simulink model "STC_Cepstral_Distance"  (Simulink 6.0)
settings: Solver=FixedStepDiscrete  SolverMode=SingleTasking  StartTime=0.0  StopTime=1  FixedStep=1/8000  RelTol=1e-3
libraries: dsplp x24, dspindex x16, dspbuff3 x8, dspsolvers x8, dspsrcs4 x6, dspsnks4 x4
settings Model: LastModifiedBy=Paulo

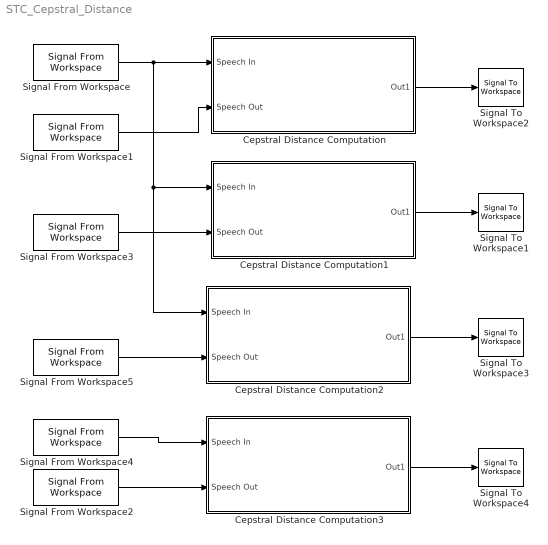
== system STC_Cepstral_Distance ==
  Cepstral Distance Computation : Subsystem
  Cepstral Distance Computation1 : Subsystem
  Cepstral Distance Computation2 : Subsystem
  Cepstral Distance Computation3 : Subsystem
  Signal From Workspace : dspsrcs4/Signal From Workspace  X=speech  Ts=1/8000  nsamps=160  OutputAfterFinalValue=Setting to zero
  Signal From Workspace1 : dspsrcs4/Signal From Workspace  X=speech1  Ts=1/8000  nsamps=160  OutputAfterFinalValue=Setting to zero
  Signal From Workspace2 : dspsrcs4/Signal From Workspace  X=speech3  Ts=1/8000  nsamps=160  OutputAfterFinalValue=Setting to zero
  Signal From Workspace3 : dspsrcs4/Signal From Workspace  X=speech2  Ts=1/8000  nsamps=160  OutputAfterFinalValue=Setting to zero
  Signal From Workspace4 : dspsrcs4/Signal From Workspace  X=residual  Ts=1/8000  nsamps=160  OutputAfterFinalValue=Setting to zero
  Signal From Workspace5 : dspsrcs4/Signal From Workspace  X=speech3  Ts=1/8000  nsamps=160  OutputAfterFinalValue=Setting to zero
  Signal To Workspace1 : dspsnks4/Signal To Workspace  VariableName=CD2  FrameMode=Concatenate frames (2-D array)
      settings: FixptAsFi=off
  Signal To Workspace2 : dspsnks4/Signal To Workspace  VariableName=CD1  FrameMode=Concatenate frames (2-D array)
      settings: FixptAsFi=off
  Signal To Workspace3 : dspsnks4/Signal To Workspace  VariableName=CD3  FrameMode=Concatenate frames (2-D array)
      settings: FixptAsFi=off
  Signal To Workspace4 : dspsnks4/Signal To Workspace  VariableName=CD4  FrameMode=Concatenate frames (2-D array)
      settings: FixptAsFi=off
  wires:
  Signal From Workspace/1 -> Cepstral Distance Computation/1(Speech In), Cepstral Distance Computation1/1(Speech In), Cepstral Distance Computation2/1(Speech In)
  Signal From Workspace1/1 -> Cepstral Distance Computation/2(Speech Out)
  Cepstral Distance Computation/1(Out1) -> Signal To Workspace2/1
  Signal From Workspace3/1 -> Cepstral Distance Computation1/2(Speech Out)
  Cepstral Distance Computation1/1(Out1) -> Signal To Workspace1/1
  Signal From Workspace5/1 -> Cepstral Distance Computation2/2(Speech Out)
  Cepstral Distance Computation2/1(Out1) -> Signal To Workspace3/1
  Signal From Workspace2/1 -> Cepstral Distance Computation3/2(Speech Out)
  Cepstral Distance Computation3/1(Out1) -> Signal To Workspace4/1
  Signal From Workspace4/1 -> Cepstral Distance Computation3/1(Speech In)

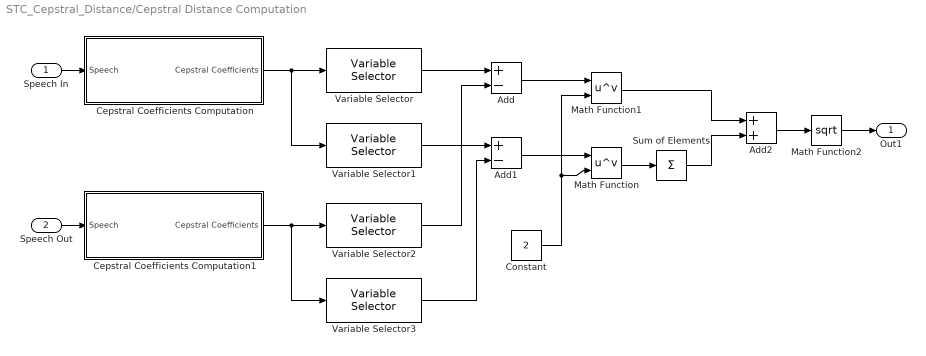
== system STC_Cepstral_Distance/Cepstral Distance Computation ==
  Speech In : Inport  Port=1  LatchInput=off
  Speech Out : Inport  Port=2  LatchInput=off
  Add : Sum  Inputs=+-  OutScaling=2^-10
  Add1 : Sum  Inputs=+-  OutScaling=2^-10
  Add2 : Sum  OutScaling=2^-10
  Cepstral Coefficients Computation : Subsystem
  Cepstral Coefficients Computation1 : Subsystem
  Constant : Constant  Value=2
  Math Function : Math  Operator=pow  SaturateOnIntegerOverflow=on
  Math Function1 : Math  Operator=pow  SaturateOnIntegerOverflow=on
  Math Function2 : Math  Operator=sqrt  SaturateOnIntegerOverflow=on
  Sum of Elements : Sum  Inputs=+  OutScaling=2^-10
  Variable Selector : dspindex/Variable Selector  rowsOrCols=Rows  IdxMode=Fixed  Elements=[1]  ZerOneIdxMode=One-based  errmode=Clip Index
  Variable Selector1 : dspindex/Variable Selector  rowsOrCols=Rows  IdxMode=Fixed  Elements=[2:21]  ZerOneIdxMode=One-based  errmode=Clip Index
  Variable Selector2 : dspindex/Variable Selector  rowsOrCols=Rows  IdxMode=Fixed  Elements=[1]  ZerOneIdxMode=One-based  errmode=Clip Index
  Variable Selector3 : dspindex/Variable Selector  rowsOrCols=Rows  IdxMode=Fixed  Elements=[2:21]  ZerOneIdxMode=One-based  errmode=Clip Index
  Out1 : Outport
  wires:
  Cepstral Coefficients Computation/1(Cepstral Coefficients) -> Variable Selector/1, Variable Selector1/1
  Cepstral Coefficients Computation1/1(Cepstral Coefficients) -> Variable Selector2/1, Variable Selector3/1
  Variable Selector/1 -> Add/1
  Variable Selector2/1 -> Add/2
  Variable Selector3/1 -> Add1/2
  Variable Selector1/1 -> Add1/1
  Add1/1 -> Math Function/1
  Constant/1 -> Math Function/2, Math Function1/2
  Math Function/1 -> Sum of Elements/1
  Add/1 -> Math Function1/1
  Sum of Elements/1 -> Add2/2
  Math Function1/1 -> Add2/1
  Add2/1 -> Math Function2/1
  Speech In/1 -> Cepstral Coefficients Computation/1(Speech)
  Math Function2/1 -> Out1/1
  Speech Out/1 -> Cepstral Coefficients Computation1/1(Speech)

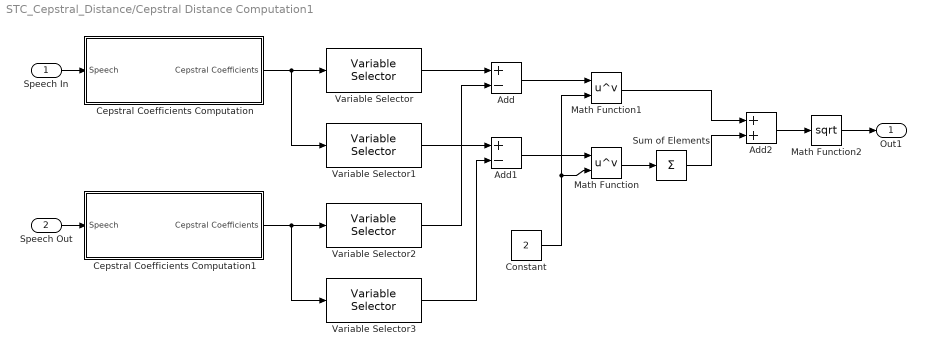
== system STC_Cepstral_Distance/Cepstral Distance Computation1 ==
  Speech In : Inport  Port=1  LatchInput=off
  Speech Out : Inport  Port=2  LatchInput=off
  Add : Sum  Inputs=+-  OutScaling=2^-10
  Add1 : Sum  Inputs=+-  OutScaling=2^-10
  Add2 : Sum  OutScaling=2^-10
  Cepstral Coefficients Computation : Subsystem
  Cepstral Coefficients Computation1 : Subsystem
  Constant : Constant  Value=2
  Math Function : Math  Operator=pow  SaturateOnIntegerOverflow=on
  Math Function1 : Math  Operator=pow  SaturateOnIntegerOverflow=on
  Math Function2 : Math  Operator=sqrt  SaturateOnIntegerOverflow=on
  Sum of Elements : Sum  Inputs=+  OutScaling=2^-10
  Variable Selector : dspindex/Variable Selector  rowsOrCols=Rows  IdxMode=Fixed  Elements=[1]  ZerOneIdxMode=One-based  errmode=Clip Index
  Variable Selector1 : dspindex/Variable Selector  rowsOrCols=Rows  IdxMode=Fixed  Elements=[2:21]  ZerOneIdxMode=One-based  errmode=Clip Index
  Variable Selector2 : dspindex/Variable Selector  rowsOrCols=Rows  IdxMode=Fixed  Elements=[1]  ZerOneIdxMode=One-based  errmode=Clip Index
  Variable Selector3 : dspindex/Variable Selector  rowsOrCols=Rows  IdxMode=Fixed  Elements=[2:21]  ZerOneIdxMode=One-based  errmode=Clip Index
  Out1 : Outport
  wires:
  Cepstral Coefficients Computation/1(Cepstral Coefficients) -> Variable Selector/1, Variable Selector1/1
  Cepstral Coefficients Computation1/1(Cepstral Coefficients) -> Variable Selector2/1, Variable Selector3/1
  Variable Selector/1 -> Add/1
  Variable Selector2/1 -> Add/2
  Variable Selector3/1 -> Add1/2
  Variable Selector1/1 -> Add1/1
  Add1/1 -> Math Function/1
  Constant/1 -> Math Function/2, Math Function1/2
  Math Function/1 -> Sum of Elements/1
  Add/1 -> Math Function1/1
  Sum of Elements/1 -> Add2/2
  Math Function1/1 -> Add2/1
  Add2/1 -> Math Function2/1
  Speech In/1 -> Cepstral Coefficients Computation/1(Speech)
  Math Function2/1 -> Out1/1
  Speech Out/1 -> Cepstral Coefficients Computation1/1(Speech)

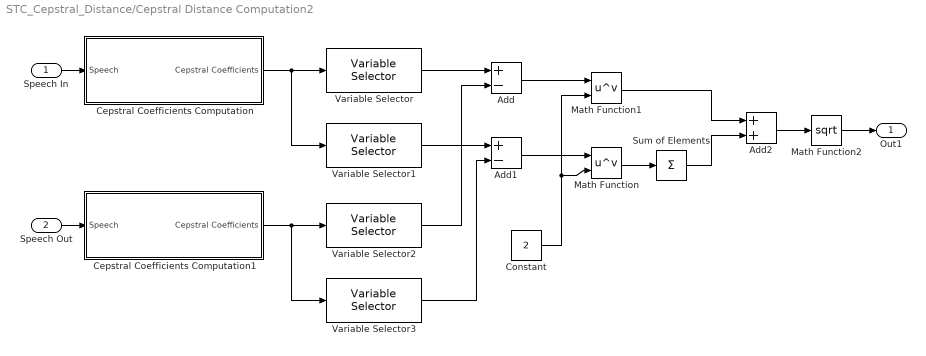
== system STC_Cepstral_Distance/Cepstral Distance Computation2 ==
  Speech In : Inport  Port=1  LatchInput=off
  Speech Out : Inport  Port=2  LatchInput=off
  Add : Sum  Inputs=+-  OutScaling=2^-10
  Add1 : Sum  Inputs=+-  OutScaling=2^-10
  Add2 : Sum  OutScaling=2^-10
  Cepstral Coefficients Computation : Subsystem
  Cepstral Coefficients Computation1 : Subsystem
  Constant : Constant  Value=2
  Math Function : Math  Operator=pow  SaturateOnIntegerOverflow=on
  Math Function1 : Math  Operator=pow  SaturateOnIntegerOverflow=on
  Math Function2 : Math  Operator=sqrt  SaturateOnIntegerOverflow=on
  Sum of Elements : Sum  Inputs=+  OutScaling=2^-10
  Variable Selector : dspindex/Variable Selector  rowsOrCols=Rows  IdxMode=Fixed  Elements=[1]  ZerOneIdxMode=One-based  errmode=Clip Index
  Variable Selector1 : dspindex/Variable Selector  rowsOrCols=Rows  IdxMode=Fixed  Elements=[2:21]  ZerOneIdxMode=One-based  errmode=Clip Index
  Variable Selector2 : dspindex/Variable Selector  rowsOrCols=Rows  IdxMode=Fixed  Elements=[1]  ZerOneIdxMode=One-based  errmode=Clip Index
  Variable Selector3 : dspindex/Variable Selector  rowsOrCols=Rows  IdxMode=Fixed  Elements=[2:21]  ZerOneIdxMode=One-based  errmode=Clip Index
  Out1 : Outport
  wires:
  Cepstral Coefficients Computation/1(Cepstral Coefficients) -> Variable Selector/1, Variable Selector1/1
  Cepstral Coefficients Computation1/1(Cepstral Coefficients) -> Variable Selector2/1, Variable Selector3/1
  Variable Selector/1 -> Add/1
  Variable Selector2/1 -> Add/2
  Variable Selector3/1 -> Add1/2
  Variable Selector1/1 -> Add1/1
  Add1/1 -> Math Function/1
  Constant/1 -> Math Function/2, Math Function1/2
  Math Function/1 -> Sum of Elements/1
  Add/1 -> Math Function1/1
  Sum of Elements/1 -> Add2/2
  Math Function1/1 -> Add2/1
  Add2/1 -> Math Function2/1
  Speech In/1 -> Cepstral Coefficients Computation/1(Speech)
  Math Function2/1 -> Out1/1
  Speech Out/1 -> Cepstral Coefficients Computation1/1(Speech)

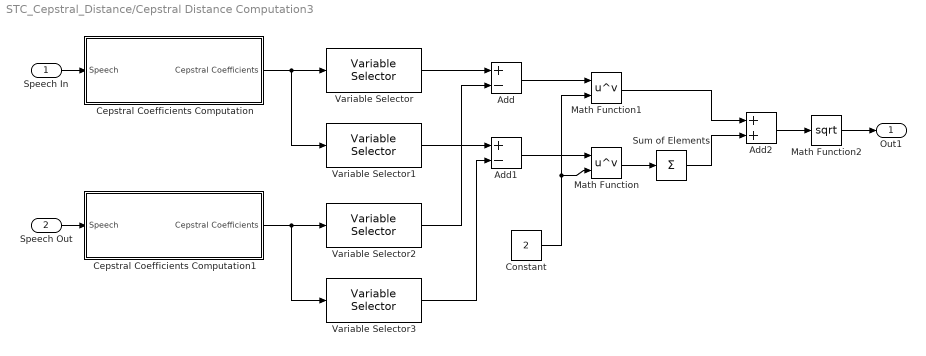
== system STC_Cepstral_Distance/Cepstral Distance Computation3 ==
  Speech In : Inport  Port=1  LatchInput=off
  Speech Out : Inport  Port=2  LatchInput=off
  Add : Sum  Inputs=+-  OutScaling=2^-10
  Add1 : Sum  Inputs=+-  OutScaling=2^-10
  Add2 : Sum  OutScaling=2^-10
  Cepstral Coefficients Computation : Subsystem
  Cepstral Coefficients Computation1 : Subsystem
  Constant : Constant  Value=2
  Math Function : Math  Operator=pow  SaturateOnIntegerOverflow=on
  Math Function1 : Math  Operator=pow  SaturateOnIntegerOverflow=on
  Math Function2 : Math  Operator=sqrt  SaturateOnIntegerOverflow=on
  Sum of Elements : Sum  Inputs=+  OutScaling=2^-10
  Variable Selector : dspindex/Variable Selector  rowsOrCols=Rows  IdxMode=Fixed  Elements=[1]  ZerOneIdxMode=One-based  errmode=Clip Index
  Variable Selector1 : dspindex/Variable Selector  rowsOrCols=Rows  IdxMode=Fixed  Elements=[2:21]  ZerOneIdxMode=One-based  errmode=Clip Index
  Variable Selector2 : dspindex/Variable Selector  rowsOrCols=Rows  IdxMode=Fixed  Elements=[1]  ZerOneIdxMode=One-based  errmode=Clip Index
  Variable Selector3 : dspindex/Variable Selector  rowsOrCols=Rows  IdxMode=Fixed  Elements=[2:21]  ZerOneIdxMode=One-based  errmode=Clip Index
  Out1 : Outport
  wires:
  Cepstral Coefficients Computation/1(Cepstral Coefficients) -> Variable Selector/1, Variable Selector1/1
  Cepstral Coefficients Computation1/1(Cepstral Coefficients) -> Variable Selector2/1, Variable Selector3/1
  Variable Selector/1 -> Add/1
  Variable Selector2/1 -> Add/2
  Variable Selector3/1 -> Add1/2
  Variable Selector1/1 -> Add1/1
  Add1/1 -> Math Function/1
  Constant/1 -> Math Function/2, Math Function1/2
  Math Function/1 -> Sum of Elements/1
  Add/1 -> Math Function1/1
  Sum of Elements/1 -> Add2/2
  Math Function1/1 -> Add2/1
  Add2/1 -> Math Function2/1
  Speech In/1 -> Cepstral Coefficients Computation/1(Speech)
  Math Function2/1 -> Out1/1
  Speech Out/1 -> Cepstral Coefficients Computation1/1(Speech)

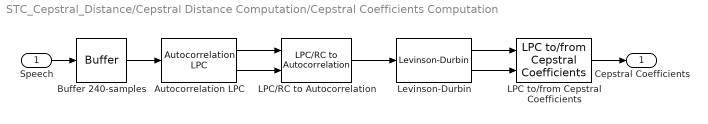
== system STC_Cepstral_Distance/Cepstral Distance Computation/Cepstral Coefficients Computation ==
  Speech : Inport  Port=1  LatchInput=off
  Autocorrelation LPC : dsplp/Autocorrelation LPC  lpcCoeffOutFcn=A  lpcOutP=on  inherit_prediction_order=off  order=10
  Buffer 240-samples : dspbuff3/Buffer  N=240  V=80  ic=0
  "LPC to/from Cepstral Coefficients " : dsplp/LPC to//from Cepstral Coefficients   conversion=LPCs to cepstral coefficients  enerpp=via input port  outpower=off  sizecb=off  nceps=21  error=Replace it with 1
  LPC/RC to Autocorrelation : dsplp/LPC//RC to Autocorrelation  conversion=LPC to autocorrelation  perr_spec=Via input port  error=Replace it with 1
  Levinson-Durbin : dspsolvers/Levinson-Durbin  DialogController=dspDDGCreate  DialogControllerArgs=DataTag0  coeffOutFcn=A  outP=on  zeroInpHandling=on  firstCoeffMode=Binary point scaling  firstCoeffWordLength=16  firstCoeffFracLength=15  secondCoeffMode=Binary point scaling  secondCoeffWordLength=16  secondCoeffFracLength=15  accumMode=Binary point scaling  accumWordLength=32  accumFracLength=30  prodOutputMode=Binary point scaling  prodOutputWordLength=32  prodOutputFracLength=30  roundingMode=Floor  overflowMode=off
      settings: allowOverrides=off
  Cepstral Coefficients : Outport
  wires:
  Autocorrelation LPC/1 -> LPC/RC to Autocorrelation/1
  Autocorrelation LPC/2 -> LPC/RC to Autocorrelation/2
  LPC/RC to Autocorrelation/1 -> Levinson-Durbin/1
  Buffer 240-samples/1 -> Autocorrelation LPC/1
  Levinson-Durbin/2 -> "LPC to/from Cepstral Coefficients "/2
  Levinson-Durbin/1 -> "LPC to/from Cepstral Coefficients "/1
  Speech/1 -> Buffer 240-samples/1
  "LPC to/from Cepstral Coefficients "/1 -> Cepstral Coefficients/1

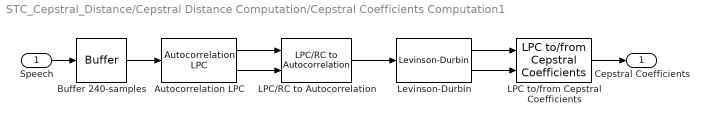
== system STC_Cepstral_Distance/Cepstral Distance Computation/Cepstral Coefficients Computation1 ==
  Speech : Inport  Port=1  LatchInput=off
  Autocorrelation LPC : dsplp/Autocorrelation LPC  lpcCoeffOutFcn=A  lpcOutP=on  inherit_prediction_order=off  order=10
  Buffer 240-samples : dspbuff3/Buffer  N=240  V=80  ic=0
  "LPC to/from Cepstral Coefficients " : dsplp/LPC to//from Cepstral Coefficients   conversion=LPCs to cepstral coefficients  enerpp=via input port  outpower=off  sizecb=off  nceps=21  error=Replace it with 1
  LPC/RC to Autocorrelation : dsplp/LPC//RC to Autocorrelation  conversion=LPC to autocorrelation  perr_spec=Via input port  error=Replace it with 1
  Levinson-Durbin : dspsolvers/Levinson-Durbin  DialogController=dspDDGCreate  DialogControllerArgs=DataTag1  coeffOutFcn=A  outP=on  zeroInpHandling=on  firstCoeffMode=Binary point scaling  firstCoeffWordLength=16  firstCoeffFracLength=15  secondCoeffMode=Binary point scaling  secondCoeffWordLength=16  secondCoeffFracLength=15  accumMode=Binary point scaling  accumWordLength=32  accumFracLength=30  prodOutputMode=Binary point scaling  prodOutputWordLength=32  prodOutputFracLength=30  roundingMode=Floor  overflowMode=off
      settings: allowOverrides=off
  Cepstral Coefficients : Outport
  wires:
  Autocorrelation LPC/1 -> LPC/RC to Autocorrelation/1
  Autocorrelation LPC/2 -> LPC/RC to Autocorrelation/2
  LPC/RC to Autocorrelation/1 -> Levinson-Durbin/1
  Buffer 240-samples/1 -> Autocorrelation LPC/1
  Levinson-Durbin/2 -> "LPC to/from Cepstral Coefficients "/2
  Levinson-Durbin/1 -> "LPC to/from Cepstral Coefficients "/1
  Speech/1 -> Buffer 240-samples/1
  "LPC to/from Cepstral Coefficients "/1 -> Cepstral Coefficients/1

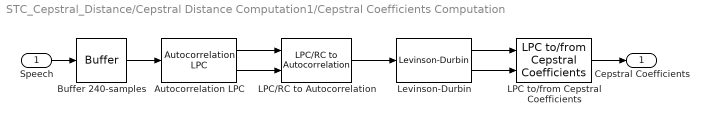
== system STC_Cepstral_Distance/Cepstral Distance Computation1/Cepstral Coefficients Computation ==
  Speech : Inport  Port=1  LatchInput=off
  Autocorrelation LPC : dsplp/Autocorrelation LPC  lpcCoeffOutFcn=A  lpcOutP=on  inherit_prediction_order=off  order=10
  Buffer 240-samples : dspbuff3/Buffer  N=240  V=80  ic=0
  "LPC to/from Cepstral Coefficients " : dsplp/LPC to//from Cepstral Coefficients   conversion=LPCs to cepstral coefficients  enerpp=via input port  outpower=off  sizecb=off  nceps=21  error=Replace it with 1
  LPC/RC to Autocorrelation : dsplp/LPC//RC to Autocorrelation  conversion=LPC to autocorrelation  perr_spec=Via input port  error=Replace it with 1
  Levinson-Durbin : dspsolvers/Levinson-Durbin  DialogController=dspDDGCreate  DialogControllerArgs=DataTag2  coeffOutFcn=A  outP=on  zeroInpHandling=on  firstCoeffMode=Binary point scaling  firstCoeffWordLength=16  firstCoeffFracLength=15  secondCoeffMode=Binary point scaling  secondCoeffWordLength=16  secondCoeffFracLength=15  accumMode=Binary point scaling  accumWordLength=32  accumFracLength=30  prodOutputMode=Binary point scaling  prodOutputWordLength=32  prodOutputFracLength=30  roundingMode=Floor  overflowMode=off
      settings: allowOverrides=off
  Cepstral Coefficients : Outport
  wires:
  Autocorrelation LPC/1 -> LPC/RC to Autocorrelation/1
  Autocorrelation LPC/2 -> LPC/RC to Autocorrelation/2
  LPC/RC to Autocorrelation/1 -> Levinson-Durbin/1
  Buffer 240-samples/1 -> Autocorrelation LPC/1
  Levinson-Durbin/2 -> "LPC to/from Cepstral Coefficients "/2
  Levinson-Durbin/1 -> "LPC to/from Cepstral Coefficients "/1
  Speech/1 -> Buffer 240-samples/1
  "LPC to/from Cepstral Coefficients "/1 -> Cepstral Coefficients/1

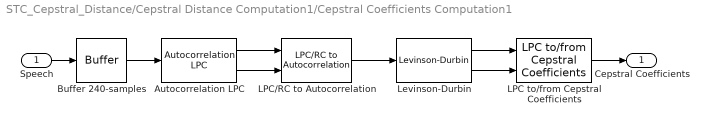
== system STC_Cepstral_Distance/Cepstral Distance Computation1/Cepstral Coefficients Computation1 ==
  Speech : Inport  Port=1  LatchInput=off
  Autocorrelation LPC : dsplp/Autocorrelation LPC  lpcCoeffOutFcn=A  lpcOutP=on  inherit_prediction_order=off  order=10
  Buffer 240-samples : dspbuff3/Buffer  N=240  V=80  ic=0
  "LPC to/from Cepstral Coefficients " : dsplp/LPC to//from Cepstral Coefficients   conversion=LPCs to cepstral coefficients  enerpp=via input port  outpower=off  sizecb=off  nceps=21  error=Replace it with 1
  LPC/RC to Autocorrelation : dsplp/LPC//RC to Autocorrelation  conversion=LPC to autocorrelation  perr_spec=Via input port  error=Replace it with 1
  Levinson-Durbin : dspsolvers/Levinson-Durbin  DialogController=dspDDGCreate  DialogControllerArgs=DataTag3  coeffOutFcn=A  outP=on  zeroInpHandling=on  firstCoeffMode=Binary point scaling  firstCoeffWordLength=16  firstCoeffFracLength=15  secondCoeffMode=Binary point scaling  secondCoeffWordLength=16  secondCoeffFracLength=15  accumMode=Binary point scaling  accumWordLength=32  accumFracLength=30  prodOutputMode=Binary point scaling  prodOutputWordLength=32  prodOutputFracLength=30  roundingMode=Floor  overflowMode=off
      settings: allowOverrides=off
  Cepstral Coefficients : Outport
  wires:
  Autocorrelation LPC/1 -> LPC/RC to Autocorrelation/1
  Autocorrelation LPC/2 -> LPC/RC to Autocorrelation/2
  LPC/RC to Autocorrelation/1 -> Levinson-Durbin/1
  Buffer 240-samples/1 -> Autocorrelation LPC/1
  Levinson-Durbin/2 -> "LPC to/from Cepstral Coefficients "/2
  Levinson-Durbin/1 -> "LPC to/from Cepstral Coefficients "/1
  Speech/1 -> Buffer 240-samples/1
  "LPC to/from Cepstral Coefficients "/1 -> Cepstral Coefficients/1

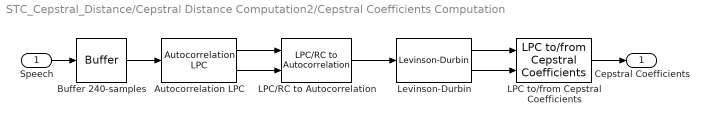
== system STC_Cepstral_Distance/Cepstral Distance Computation2/Cepstral Coefficients Computation ==
  Speech : Inport  Port=1  LatchInput=off
  Autocorrelation LPC : dsplp/Autocorrelation LPC  lpcCoeffOutFcn=A  lpcOutP=on  inherit_prediction_order=off  order=10
  Buffer 240-samples : dspbuff3/Buffer  N=240  V=80  ic=0
  "LPC to/from Cepstral Coefficients " : dsplp/LPC to//from Cepstral Coefficients   conversion=LPCs to cepstral coefficients  enerpp=via input port  outpower=off  sizecb=off  nceps=21  error=Replace it with 1
  LPC/RC to Autocorrelation : dsplp/LPC//RC to Autocorrelation  conversion=LPC to autocorrelation  perr_spec=Via input port  error=Replace it with 1
  Levinson-Durbin : dspsolvers/Levinson-Durbin  DialogController=dspDDGCreate  DialogControllerArgs=DataTag4  coeffOutFcn=A  outP=on  zeroInpHandling=on  firstCoeffMode=Binary point scaling  firstCoeffWordLength=16  firstCoeffFracLength=15  secondCoeffMode=Binary point scaling  secondCoeffWordLength=16  secondCoeffFracLength=15  accumMode=Binary point scaling  accumWordLength=32  accumFracLength=30  prodOutputMode=Binary point scaling  prodOutputWordLength=32  prodOutputFracLength=30  roundingMode=Floor  overflowMode=off
      settings: allowOverrides=off
  Cepstral Coefficients : Outport
  wires:
  Autocorrelation LPC/1 -> LPC/RC to Autocorrelation/1
  Autocorrelation LPC/2 -> LPC/RC to Autocorrelation/2
  LPC/RC to Autocorrelation/1 -> Levinson-Durbin/1
  Buffer 240-samples/1 -> Autocorrelation LPC/1
  Levinson-Durbin/2 -> "LPC to/from Cepstral Coefficients "/2
  Levinson-Durbin/1 -> "LPC to/from Cepstral Coefficients "/1
  Speech/1 -> Buffer 240-samples/1
  "LPC to/from Cepstral Coefficients "/1 -> Cepstral Coefficients/1

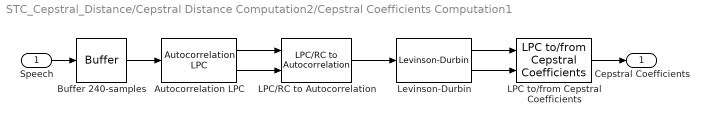
== system STC_Cepstral_Distance/Cepstral Distance Computation2/Cepstral Coefficients Computation1 ==
  Speech : Inport  Port=1  LatchInput=off
  Autocorrelation LPC : dsplp/Autocorrelation LPC  lpcCoeffOutFcn=A  lpcOutP=on  inherit_prediction_order=off  order=10
  Buffer 240-samples : dspbuff3/Buffer  N=240  V=80  ic=0
  "LPC to/from Cepstral Coefficients " : dsplp/LPC to//from Cepstral Coefficients   conversion=LPCs to cepstral coefficients  enerpp=via input port  outpower=off  sizecb=off  nceps=21  error=Replace it with 1
  LPC/RC to Autocorrelation : dsplp/LPC//RC to Autocorrelation  conversion=LPC to autocorrelation  perr_spec=Via input port  error=Replace it with 1
  Levinson-Durbin : dspsolvers/Levinson-Durbin  DialogController=dspDDGCreate  DialogControllerArgs=DataTag5  coeffOutFcn=A  outP=on  zeroInpHandling=on  firstCoeffMode=Binary point scaling  firstCoeffWordLength=16  firstCoeffFracLength=15  secondCoeffMode=Binary point scaling  secondCoeffWordLength=16  secondCoeffFracLength=15  accumMode=Binary point scaling  accumWordLength=32  accumFracLength=30  prodOutputMode=Binary point scaling  prodOutputWordLength=32  prodOutputFracLength=30  roundingMode=Floor  overflowMode=off
      settings: allowOverrides=off
  Cepstral Coefficients : Outport
  wires:
  Autocorrelation LPC/1 -> LPC/RC to Autocorrelation/1
  Autocorrelation LPC/2 -> LPC/RC to Autocorrelation/2
  LPC/RC to Autocorrelation/1 -> Levinson-Durbin/1
  Buffer 240-samples/1 -> Autocorrelation LPC/1
  Levinson-Durbin/2 -> "LPC to/from Cepstral Coefficients "/2
  Levinson-Durbin/1 -> "LPC to/from Cepstral Coefficients "/1
  Speech/1 -> Buffer 240-samples/1
  "LPC to/from Cepstral Coefficients "/1 -> Cepstral Coefficients/1

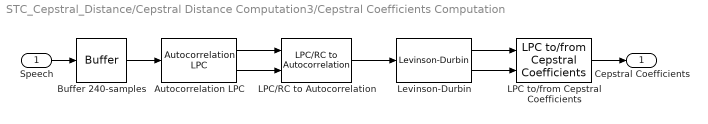
== system STC_Cepstral_Distance/Cepstral Distance Computation3/Cepstral Coefficients Computation ==
  Speech : Inport  Port=1  LatchInput=off
  Autocorrelation LPC : dsplp/Autocorrelation LPC  lpcCoeffOutFcn=A  lpcOutP=on  inherit_prediction_order=off  order=10
  Buffer 240-samples : dspbuff3/Buffer  N=240  V=80  ic=0
  "LPC to/from Cepstral Coefficients " : dsplp/LPC to//from Cepstral Coefficients   conversion=LPCs to cepstral coefficients  enerpp=via input port  outpower=off  sizecb=off  nceps=21  error=Replace it with 1
  LPC/RC to Autocorrelation : dsplp/LPC//RC to Autocorrelation  conversion=LPC to autocorrelation  perr_spec=Via input port  error=Replace it with 1
  Levinson-Durbin : dspsolvers/Levinson-Durbin  DialogController=dspDDGCreate  DialogControllerArgs=DataTag6  coeffOutFcn=A  outP=on  zeroInpHandling=on  firstCoeffMode=Binary point scaling  firstCoeffWordLength=16  firstCoeffFracLength=15  secondCoeffMode=Binary point scaling  secondCoeffWordLength=16  secondCoeffFracLength=15  accumMode=Binary point scaling  accumWordLength=32  accumFracLength=30  prodOutputMode=Binary point scaling  prodOutputWordLength=32  prodOutputFracLength=30  roundingMode=Floor  overflowMode=off
      settings: allowOverrides=off
  Cepstral Coefficients : Outport
  wires:
  Autocorrelation LPC/1 -> LPC/RC to Autocorrelation/1
  Autocorrelation LPC/2 -> LPC/RC to Autocorrelation/2
  LPC/RC to Autocorrelation/1 -> Levinson-Durbin/1
  Buffer 240-samples/1 -> Autocorrelation LPC/1
  Levinson-Durbin/2 -> "LPC to/from Cepstral Coefficients "/2
  Levinson-Durbin/1 -> "LPC to/from Cepstral Coefficients "/1
  Speech/1 -> Buffer 240-samples/1
  "LPC to/from Cepstral Coefficients "/1 -> Cepstral Coefficients/1

== system STC_Cepstral_Distance/Cepstral Distance Computation3/Cepstral Coefficients Computation1 ==
  Speech : Inport  Port=1  LatchInput=off
  Autocorrelation LPC : dsplp/Autocorrelation LPC  lpcCoeffOutFcn=A  lpcOutP=on  inherit_prediction_order=off  order=10
  Buffer 240-samples : dspbuff3/Buffer  N=240  V=80  ic=0
  "LPC to/from Cepstral Coefficients " : dsplp/LPC to//from Cepstral Coefficients   conversion=LPCs to cepstral coefficients  enerpp=via input port  outpower=off  sizecb=off  nceps=21  error=Replace it with 1
  LPC/RC to Autocorrelation : dsplp/LPC//RC to Autocorrelation  conversion=LPC to autocorrelation  perr_spec=Via input port  error=Replace it with 1
  Levinson-Durbin : dspsolvers/Levinson-Durbin  DialogController=dspDDGCreate  DialogControllerArgs=DataTag7  coeffOutFcn=A  outP=on  zeroInpHandling=on  firstCoeffMode=Binary point scaling  firstCoeffWordLength=16  firstCoeffFracLength=15  secondCoeffMode=Binary point scaling  secondCoeffWordLength=16  secondCoeffFracLength=15  accumMode=Binary point scaling  accumWordLength=32  accumFracLength=30  prodOutputMode=Binary point scaling  prodOutputWordLength=32  prodOutputFracLength=30  roundingMode=Floor  overflowMode=off
      settings: allowOverrides=off
  Cepstral Coefficients : Outport
  wires:
  Autocorrelation LPC/1 -> LPC/RC to Autocorrelation/1
  Autocorrelation LPC/2 -> LPC/RC to Autocorrelation/2
  LPC/RC to Autocorrelation/1 -> Levinson-Durbin/1
  Buffer 240-samples/1 -> Autocorrelation LPC/1
  Levinson-Durbin/2 -> "LPC to/from Cepstral Coefficients "/2
  Levinson-Durbin/1 -> "LPC to/from Cepstral Coefficients "/1
  Speech/1 -> Buffer 240-samples/1
  "LPC to/from Cepstral Coefficients "/1 -> Cepstral Coefficients/1
